simulink model "SS_task9"  (R2021b)
settings: Solver=FixedStepAuto  StartTime=0.0  StopTime=10.0  FixedStep=0.01  RelTol=1e-3
values from neighbouring files (symbols this model uses):
  A_veh_sh = [0 1 0 0 ... (first row only)    [vehicle_control.m]
  A_veh_sh_cl = [0   1    0     0 ... (first row only)    [vehicle_control.m]
  B_veh_sh = [ 0 0 0 0 ... (first row only)    [vehicle_control.m]
  B_veh_sh_cl = [0 0; k1/m k2/m;0 0 ;-k1*L1/J k2*L2/J]    [vehicle_control.m]
  c_chi = 8e5    (= 800000)    [vehicle_control.m]
  C_veh_sh = [0 1 0 0;0 0 0 1]    [vehicle_control.m]
  C_veh_sh_cl = [1 0 0 0; 0 0 1 0]    [vehicle_control.m]
  cz = 15e4    (= 150000)    [vehicle_control.m]
  D_veh_sh = [0 0 0 0;0 0 0 0]    [vehicle_control.m]
  D_veh_sh_cl = [0 0; 0 0]    [vehicle_control.m]
  L1 = L    (= 6)    [vehicle_control.m]
  L2 = L    (= 6)    [vehicle_control.m]
undefined symbols (not defined in the file or in its folder): sigbuilder_block
settings Model: Creator=rivaa  LastModifiedBy=rivaa

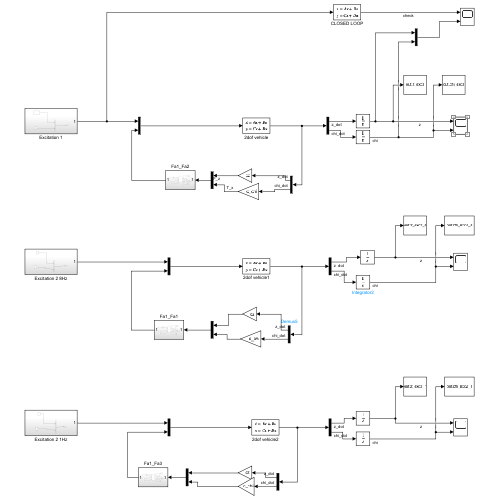
[thumbnail: Simulink's stored preview of the top-level diagram]
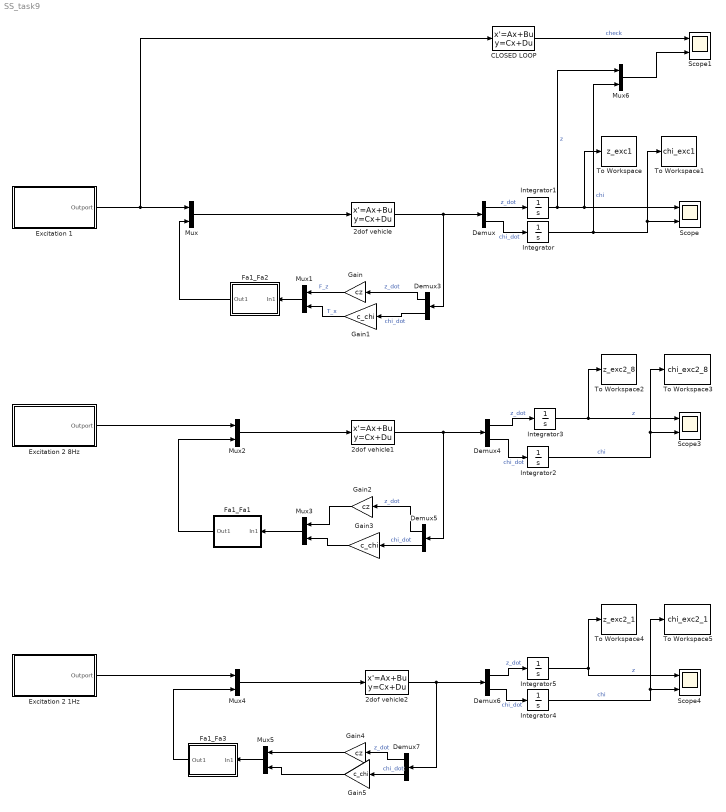
== system SS_task9 ==
  2dof vehicle : StateSpace  A=A_veh_sh  B=B_veh_sh  C=C_veh_sh  D=D_veh_sh  InitialCondition=0
  2dof vehicle1 : StateSpace  A=A_veh_sh  B=B_veh_sh  C=C_veh_sh  D=D_veh_sh  InitialCondition=0
  2dof vehicle2 : StateSpace  A=A_veh_sh  B=B_veh_sh  C=C_veh_sh  D=D_veh_sh  InitialCondition=0
  CLOSED LOOP : StateSpace  A=A_veh_sh_cl  B=B_veh_sh_cl  C=C_veh_sh_cl  D=D_veh_sh_cl  InitialCondition=0
  Demux{,3..7} (6 alike) : Demux  Outputs=2
  Excitation 1 : Subsystem
  Excitation 2 1Hz : Subsystem
  Excitation 2 8Hz : Subsystem
  Fa1_Fa1 : Subsystem
  Fa1_Fa2 : Subsystem
  Fa1_Fa3 : Subsystem
  Gain : Gain  Gain=cz
  Gain1 : Gain  Gain=c_chi
  Gain2 : Gain  Gain=cz
  Gain3 : Gain  Gain=c_chi
  Gain4 : Gain  Gain=cz
  Gain5 : Gain  Gain=c_chi
  Integrator{,1..5} (6 alike) : Integrator
  Mux{,1..6} (7 alike) : Mux  Inputs=2
  Scope{,1,3..4} (4 alike) : Scope  NumInputPorts=2
  To Workspace : ToWorkspace  VariableName=z_exc1  SampleTime=-1
      settings: Save2DSignal=2-D array (concatenate along first dimension)
  To Workspace1 : ToWorkspace  VariableName=chi_exc1  SampleTime=-1
      settings: Save2DSignal=2-D array (concatenate along first dimension)
  To Workspace2 : ToWorkspace  VariableName=z_exc2_8  SampleTime=-1
      settings: Save2DSignal=2-D array (concatenate along first dimension)
  To Workspace3 : ToWorkspace  VariableName=chi_exc2_8  SampleTime=-1
      settings: Save2DSignal=2-D array (concatenate along first dimension)
  To Workspace4 : ToWorkspace  VariableName=z_exc2_1  SampleTime=-1
      settings: Save2DSignal=2-D array (concatenate along first dimension)
  To Workspace5 : ToWorkspace  VariableName=chi_exc2_1  SampleTime=-1
      settings: Save2DSignal=2-D array (concatenate along first dimension)
  wires:
  Integrator1/1 -> Mux6/1, Scope/1, To Workspace/1  "z"
  Integrator/1 -> To Workspace1/1, Scope/2, Mux6/2  "chi"
  Mux/1 -> 2dof vehicle/1
  2dof vehicle/1 -> Demux/1, Demux3/1
  Demux3/1 -> Gain/1  "z_dot"
  Demux3/2 -> Gain1/1  "chi_dot"
  Gain/1 -> Mux1/1  "F_z"
  Gain1/1 -> Mux1/2  "T_x"
  Excitation 1/1(Outport) -> Mux/1, CLOSED LOOP/1
  Demux/2 -> Integrator/1  "chi_dot"
  Demux/1 -> Integrator1/1  "z_dot"
  Demux4/1 -> Integrator3/1  "z_dot"
  Demux4/2 -> Integrator2/1  "chi_dot"
  Excitation 2 8Hz/1(Outport) -> Mux2/1
  Gain3/1 -> Mux3/2
  Gain2/1 -> Mux3/1
  Demux5/2 -> Gain3/1  "chi_dot"
  Demux5/1 -> Gain2/1  "z_dot"
  2dof vehicle1/1 -> Demux5/1, Demux4/1
  Mux2/1 -> 2dof vehicle1/1
  Integrator2/1 -> To Workspace3/1, Scope3/2  "chi"
  Integrator3/1 -> Scope3/1, To Workspace2/1  "z"
  Integrator5/1 -> Scope4/1, To Workspace4/1  "z"
  Integrator4/1 -> To Workspace5/1, Scope4/2  "chi"
  Mux4/1 -> 2dof vehicle2/1
  2dof vehicle2/1 -> Demux6/1, Demux7/1
  Demux7/1 -> Gain4/1  "z_dot"
  Demux7/2 -> Gain5/1  "chi_dot"
  Gain4/1 -> Mux5/1
  Excitation 2 1Hz/1(Outport) -> Mux4/1
  Demux6/2 -> Integrator4/1  "chi_dot"
  Demux6/1 -> Integrator5/1  "z_dot"
  Mux1/1 -> Fa1_Fa2/1(In1)
  Fa1_Fa2/1(Out1) -> Mux/2
  Mux3/1 -> Fa1_Fa1/1(In1)
  Mux5/1 -> Fa1_Fa3/1(In1)
  Fa1_Fa3/1(Out1) -> Mux4/2
  CLOSED LOOP/1 -> Scope1/1  "check"
  Mux6/1 -> Scope1/2
  Fa1_Fa1/1(Out1) -> Mux2/2
  Gain5/1 -> Mux5/2

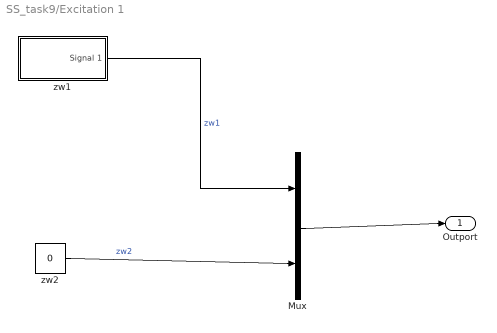
== system SS_task9/Excitation 1 ==
  Mux : Mux  Inputs=2
  zw1 : Subsystem  Tag=STV Subsys  LoadFcn=sigbuilder_block('load');  StartFcn=sigbuilder_block('start');  StopFcn=sigbuilder_block('stop');  ClipboardFcn=sigbuilder_block('clipboard');  mask(Sigbuilder block){tuvar=[0:10]}
      mask help: Simulink:masks:SigbuilderBlock_MD
      mask init:
      | if ~strcmp(get_param(bdroot(gcbh),'SimulationStatus'),'stopped') tuvar = sigbuilder_block('maskInit'); end
      settings: CopyFcn=sigbuilder_block('copy');  DeleteFcn=sigbuilder_block('delete');  ModelCloseFcn=sigbuilder_block('modelClose');  PreSaveFcn=sigbuilder_block('preSave');  PauseFcn=sigbuilder_block('pause');  ContinueFcn=sigbuilder_block('continue');  NameChangeFcn=sigbuilder_block('namechange');  OpenFcn=sigbuilder_block('open',[437.6 199.2 550.4 400 ]);  CloseFcn=sigbuilder_block('close');
      mask Display: plot(0, 0, 100, 100,[2, 2, 32, 32, 2], [68, 8, 8, 68, 68],[32, 2], [38, 38], [32, 19, 2],[53, 60, 44], [32, 17, 17, 2],[16, 16, 31, 31]);txt = getActiveGroup(gcbh);text(2, 100, txt,'verticalAlignment', 'top');
  zw2 : Constant  Value=0
  Outport : Outport
  wires:
  zw1/1(Signal 1) -> Mux/1  "zw1"
  Mux/1 -> Outport/1
  zw2/1 -> Mux/2  "zw2"

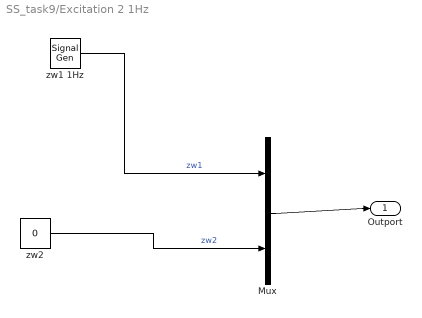
== system SS_task9/Excitation 2 1Hz ==
  Mux : Mux  Inputs=2
  zw1 1Hz : SignalGenerator  Amplitude=0.01  Frequency=2*pi*1  Units=rad/sec
  zw2 : Constant  Value=0
  Outport : Outport
  wires:
  zw2/1 -> Mux/2  "zw2"
  zw1 1Hz/1 -> Mux/1  "zw1"
  Mux/1 -> Outport/1

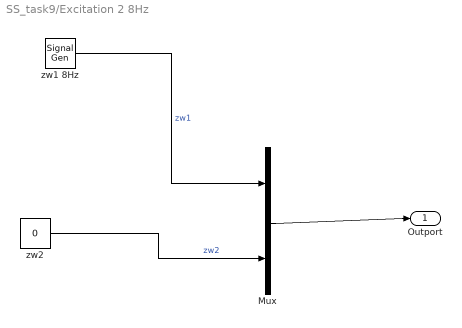
== system SS_task9/Excitation 2 8Hz ==
  Mux : Mux  Inputs=2
  zw1 8Hz : SignalGenerator  Amplitude=0.01  Frequency=2*pi*8  Units=rad/sec
  zw2 : Constant  Value=0
  Outport : Outport
  wires:
  zw2/1 -> Mux/2  "zw2"
  zw1 8Hz/1 -> Mux/1  "zw1"
  Mux/1 -> Outport/1

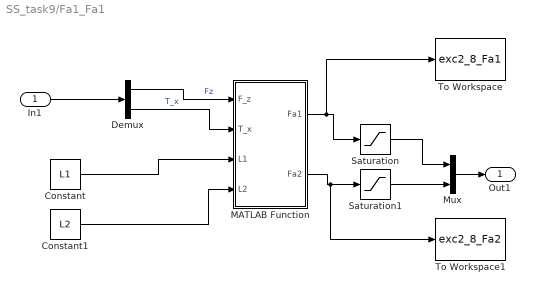
== system SS_task9/Fa1_Fa1 ==
  In1 : Inport
  Constant : Constant  Value=L1
  Constant1 : Constant  Value=L2
  Demux : Demux  Outputs=2
  MATLAB Function : MATLAB Function  TreatAsAtomicUnit=on
  Mux : Mux  Inputs=2
  Saturation : Saturate  UpperLimit=10e3  LowerLimit=-10e3
  Saturation1 : Saturate  UpperLimit=10e3  LowerLimit=-10e3
  To Workspace : ToWorkspace  VariableName=exc2_8_Fa1  SampleTime=-1
      settings: Save2DSignal=2-D array (concatenate along first dimension)
  To Workspace1 : ToWorkspace  VariableName=exc2_8_Fa2  SampleTime=-1
      settings: Save2DSignal=2-D array (concatenate along first dimension)
  Out1 : Outport
  wires:
  Saturation1/1 -> Mux/2
  Saturation/1 -> Mux/1
  MATLAB Function/2(Fa2) -> To Workspace1/1, Saturation1/1
  MATLAB Function/1(Fa1) -> To Workspace/1, Saturation/1
  Constant1/1 -> MATLAB Function/4(L2)
  Constant/1 -> MATLAB Function/3(L1)
  Demux/2 -> MATLAB Function/2(T_x)  "T_x"
  Demux/1 -> MATLAB Function/1(F_z)  "Fz"
  Mux/1 -> Out1/1
  In1/1 -> Demux/1

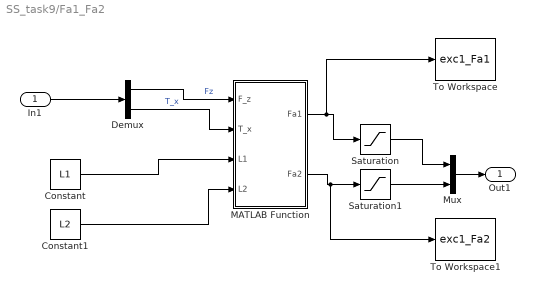
== system SS_task9/Fa1_Fa2 ==
  In1 : Inport
  Constant : Constant  Value=L1
  Constant1 : Constant  Value=L2
  Demux : Demux  Outputs=2
  MATLAB Function : MATLAB Function  TreatAsAtomicUnit=on
  Mux : Mux  Inputs=2
  Saturation : Saturate  UpperLimit=10e3  LowerLimit=-10e3
  Saturation1 : Saturate  UpperLimit=10e3  LowerLimit=-10e3
  To Workspace : ToWorkspace  VariableName=exc1_Fa1  SampleTime=-1
      settings: Save2DSignal=2-D array (concatenate along first dimension)
  To Workspace1 : ToWorkspace  VariableName=exc1_Fa2  SampleTime=-1
      settings: Save2DSignal=2-D array (concatenate along first dimension)
  Out1 : Outport
  wires:
  In1/1 -> Demux/1
  Mux/1 -> Out1/1
  Demux/1 -> MATLAB Function/1(F_z)  "Fz"
  Demux/2 -> MATLAB Function/2(T_x)  "T_x"
  Constant/1 -> MATLAB Function/3(L1)
  Constant1/1 -> MATLAB Function/4(L2)
  MATLAB Function/1(Fa1) -> To Workspace/1, Saturation/1
  MATLAB Function/2(Fa2) -> To Workspace1/1, Saturation1/1
  Saturation/1 -> Mux/1
  Saturation1/1 -> Mux/2

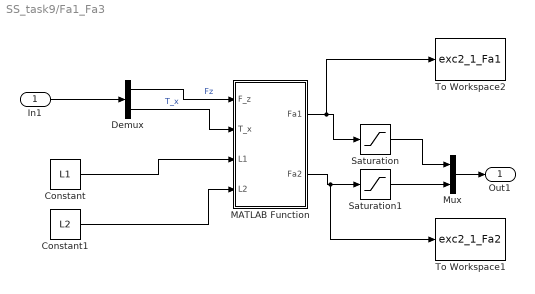
== system SS_task9/Fa1_Fa3 ==
  In1 : Inport
  Constant : Constant  Value=L1
  Constant1 : Constant  Value=L2
  Demux : Demux  Outputs=2
  MATLAB Function : MATLAB Function  TreatAsAtomicUnit=on
  Mux : Mux  Inputs=2
  Saturation : Saturate  UpperLimit=10e3  LowerLimit=-10e3
  Saturation1 : Saturate  UpperLimit=10e3  LowerLimit=-10e3
  To Workspace1 : ToWorkspace  VariableName=exc2_1_Fa2  SampleTime=-1
      settings: Save2DSignal=2-D array (concatenate along first dimension)
  To Workspace2 : ToWorkspace  VariableName=exc2_1_Fa1  SampleTime=-1
      settings: Save2DSignal=2-D array (concatenate along first dimension)
  Out1 : Outport
  wires:
  In1/1 -> Demux/1
  Mux/1 -> Out1/1
  Demux/1 -> MATLAB Function/1(F_z)  "Fz"
  Demux/2 -> MATLAB Function/2(T_x)  "T_x"
  Constant/1 -> MATLAB Function/3(L1)
  Constant1/1 -> MATLAB Function/4(L2)
  MATLAB Function/1(Fa1) -> To Workspace2/1, Saturation/1
  MATLAB Function/2(Fa2) -> To Workspace1/1, Saturation1/1
  Saturation/1 -> Mux/1
  Saturation1/1 -> Mux/2

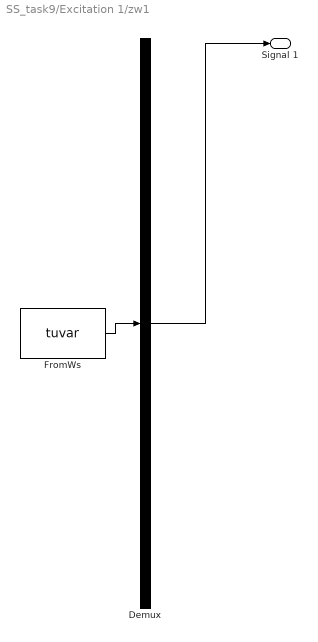
== system SS_task9/Excitation 1/zw1 ==
  Demux : Demux  Tag=STV Demux  Outputs=1
      settings: DisplayOption=none
  FromWs : FromWorkspace  Tag=STV FromWs  VariableName=tuvar
      SigBuilderData=|
      | common.afterFinalStr = 'Extrapolate'
      | common.sampleTime = 0
      | dataSet.timeRange = [0 10]
      | dataSet.name = 'Group 1'
      | sbobj.Groups.Name = 'Group 1'
      | sbobj.Groups.Signals.Name = 'Signal 1'
      | sbobj.Groups.Signals.XData = [0 0.1 0.1 10]
      | sbobj.Groups.Signals.YData = [0.03 0.03 0 0]
  Signal 1 : Outport  Tag=STV Outport
  wires:
  Demux/1 -> Signal 1/1
  FromWs/1 -> Demux/1

== matlab function SS_task9/Fa1_Fa1/MATLAB Function ==
  data: F_z input; Fa1 output; T_x input; Fa2 output; L1 input; L2 input
function [Fa1,Fa2] = fcn(F_z,T_x,L1,L2)
  Fa1 = (-T_x+F_z*L2)/(L1+L2);
  Fa2 = (T_x+F_z*L1)/(L1+L2);

== matlab function SS_task9/Fa1_Fa2/MATLAB Function ==
  data: F_z input; Fa1 output; T_x input; Fa2 output; L1 input; L2 input
function [Fa1,Fa2] = fcn(F_z,T_x,L1,L2)
  Fa1 = (-T_x+F_z*L2)/(L1+L2);
  Fa2 = (T_x+F_z*L1)/(L1+L2);

== matlab function SS_task9/Fa1_Fa3/MATLAB Function ==
  data: F_z input; Fa1 output; T_x input; Fa2 output; L1 input; L2 input
function [Fa1,Fa2] = fcn(F_z,T_x,L1,L2)
  Fa1 = (-T_x+F_z*L2)/(L1+L2);
  Fa2 = (T_x+F_z*L1)/(L1+L2);
